simulink model "LF_AC29bus_HVDCdemo_V2_1"  (R2019b)
settings: Solver=FixedStepDiscrete  StartTime=0.0  StopTime=fix(6/Ts)*Ts  FixedStep=Ts  RelTol=1e-3
InitFcn:
  | Ts_avg=150e-6;
  | Ts=50e-6;
  | 
  | %Tc_stab = 1/60/5;
  | %Tc_stab = 2/60;
  | Tc_stab = Ts;
  | 
  | 
  | Ts_avg=150e-6;
  | 
  | Ts=50e-6;
  | 
  | % Rectifier AC side :
  | VLL_nom_R = 735e3; % V
  | Fnom_R = 60;           % Hz
  | 
  | % Inverter AC side :
  | VLL_nom_I = 735e3; % V
  | Fnom_I = 60;           % Hz
  | 
  | % DC :
  | Vdc_nom = 500e3;   % V
  | Idc_nom  = 2000;     % A
undefined symbols (not defined in the file): D1, D11, Delta, test_alpha
libraries: powerlib x223, powerlib_meascontrol x57, simulink x22, sps_avr x7
(part 1 of 10)
Description:
  | Copyright 2008-2012 The MathWorks, Inc.
settings Model: SimulationMode=accelerator  Creator=MathWorks  LastModifiedBy=bhisma
settings DataIOCC: SaveFormat=StructureWithTime  SignalLoggingSaveFormat=ModelDataLogs  SaveOutput=off  SignalLogging=off  DSMLogging=off  SaveTime=off  ReturnWorkspaceOutputs=off
settings OptimizationCC: ExpressionDepthLimit=2147483647  LifeSpan=inf
settings DebuggingCC: UnderspecifiedInitializationDetection=Classic  MergeDetectMultiDrivingBlocksExec=none  SolverPrmCheckMsg=warning  FcnCallInpInsideContextMsg=warning  UnconnectedInputMsg=none  UnconnectedOutputMsg=none  UnconnectedLineMsg=none  StateNameClashWarn=warning  SFUnexpectedBacktrackingDiag=warning  SFNoUnconditionalDefaultTransitionDiag=warning  SFExecutionAtInitializationDiag=none  ArithmeticOperatorsInVariantConditions=warning
settings HardwareCC: ProdBitPerPointer=32  ProdBitPerSizeT=32  ProdBitPerPtrDiffT=32  ProdLargestAtomicFloat=None  ProdIntDivRoundTo=Undefined  ProdEndianess=Unspecified  ProdWordSize=32  ProdHWDeviceType=32-bit Generic
settings ModelReferenceCC: PropagateSignalLabelsOutOfModel=off
settings SFSimCC: SimUseLocalCustomCode=off  CustomCodeUndefinedFunction=UseInterfaceOnly
settings RTWCC: RTWUseLocalCustomCode=off
settings CodeAppCC: StateflowObjectComments=on
settings GRTTargetCC: TargetLangStandard=C89/C90 (ANSI)  GeneratePreprocessorConditionals=Disable all  CombineOutputUpdateFcns=off  GRTInterface=on
settings ConfigComp: CovMetricSettings=dw  CovHtmlReporting=on  CovSaveCumulativeToWorkspaceVar=on  CovSaveSingleToWorkspaceVar=on  CovExternalEMLEnable=off  CovSFcnEnable=off
settings SimscapeCC: SimscapeNormalizeSystem=off

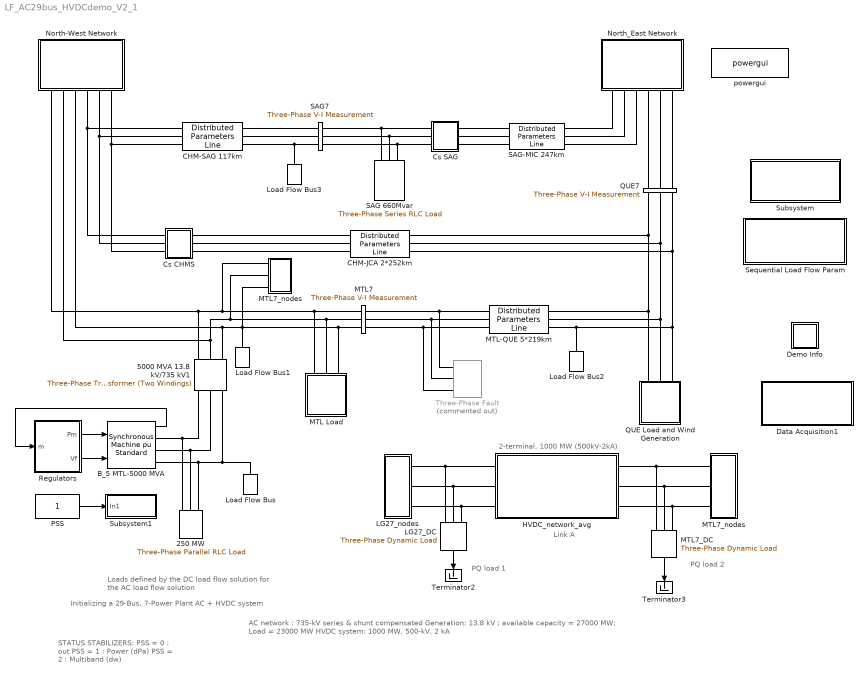
== system LF_AC29bus_HVDCdemo_V2_1 ==
  note: PQ load 1
  note: Link A
  note: AC network :  735-kV series & shunt compensated
      |               Generation: 13.8 kV ; available capacity = 27000 MW;
      |               Load = 23000 MW
      | HVDC system:  1000 MW, 500-kV, 2 kA
  note: Initializing a 29-Bus, 7-Power Plant AC + HVDC system
  note: STATUS STABILIZERS:
      | PSS = 0 :  out
      | PSS = 1 :  Power (dPa)
      | PSS = 2 :  Multiband (dw)
  note: Loads defined by the DC load flow solution
      | for the AC load flow solution
  note: 2-terminal, 1000 MW (500kV-2kA)
  note: PQ load 2
  250 MW : powerlib/Elements/Three-Phase Parallel RLC Load  LConnTagsString=A|B|C  Configuration=Y (grounded)  NominalVoltage=(13800)*1  Vabc=[1e3 1e3 1e3]  Vabcp=[1e3 1e3 1e3]  NominalFrequency=60  UnbalancedPower=off  ActivePower=250000000  InductivePower=0  CapacitivePower=0  Pabc=[10e3 9e3 11e3]  QLabc=[100 90 110]  QCabc=[100 90 110]  Pabcp=[10e3 9e3 11e3]  QLabcp=[100 90 110]  QCabcp=[100 90 110]  Measurements=None  LoadType=constant PQ
      settings: SourceProductName=Simscape Electrical
  5000 MVA 13.8 kV/735 kV1 : powerlib/Elements/Three-Phase Transformer (Two Windings)  Winding1Connection=Delta (D1)  Winding2Connection=Yg  CoreType=Three single-phase transformers  SetSaturation=off  Hysteresis=off  DataFile='basic_model'  SetInitialFlux=off  Measurements=None  UNITS=pu  NominalPower=[ 5000e6 60 ]  Winding1="[ 13.8e3 0.002  0.0]"  Winding2=[ 735e3 0.002 0.12]  Rm=500  Lm=500  L0=0.5  Saturation="[ 0,0  ;  0.005,1.2  ;  1.0,1.4 ]"  InitialFluxes=[ 0.8 , -0.8 , 0.7 ]  BreakLoop=off  DiscreteSolver=Trapezoidal iterative  DataType=off  TransfoNumber=0
      settings: SourceProductName=Simscape Electrical
  B_5 MTL-5000 MVA : powerlib/Machines/Synchronous Machine pu Standard  PresetModel=No  MechanicalLoad=Mechanical power Pm  ShowDetailedParameters=on  RotorType=Salient-pole  Units=per unit standard parameters  MeasurementBus=off  NominalParameters="[5000E6  13800   60 ]"  Reactances1=[ 31 32 33 34 35 36 37 ]  Reactances2=[ 1.305, 0.296, 0.252, 0.474, 0.243, 0.18 ]  dAxisTimeConstants=Short-circuit  qAxisTimeConstants=Open-circuit  TimeConstants1=[]  TimeConstants2=[]  TimeConstants3=[]  TimeConstants4=[]  TimeConstants5=[ 1.01, 0.053, 0.1 ]  TimeConstants6=[]  TimeConstants7=[]  TimeConstants8=[]  StatorResistance=2.8544e-3  Mechanical="[ 3.7 0  32]"  PolePairs=32  InitialConditions=[0 -107.642 0.935091 0.935091 0.935091 -27.7385 -147.738 92.2615 1.11655]  SetSaturation=off  Saturation=[0.6404,0.7127,0.8441,0.9214,0.9956,1.082,1.19,1.316,1.457;0.7,0.7698,0.8872,0.9466,0.9969,1.046,1.1,1.151,1.201]  LoadFlowParameters=[1 4000000000 0 0 0]  TsPowergui=0  TsBlock=-1  IterativeModel=Trapezoidal non iterative  IterativeDiscreteModel=Trapezoidal non iterative  BusType=PV  Pref=4500000000  Qref=0  Qmin=-Inf  Qmax=Inf  PLF=0  QLF=0
      settings: AttributesFormatString=\n\n  SourceProductName=Simscape Electrical
  CHM-JCA 2*252km : powerlib/Elements/Distributed Parameters Line  Phases=3  Frequency=60  Resistance="[0.01273  0.3864]/2"  Inductance="[0.9337e-3  4.1264e-3]/2"  Capacitance=[12.74e-9 7.751e-9]*2  Length=252  x1=[-0.00145 1.55144717799976e-09 0 0;-0.0014 1.46301284014983e-09 0 0;-0.00135 1.3740587008041e-09 0 0;-0.0013 1.28461636494472e-09 0 0;-0.00125 1.19471761100772e-09 0 0;-0.0012 1.10439437959232e-09 0 0;-0.00115 1.01367876211256e-09 0 0;-0.0011 9.22602989395366e-10 0 0;-0.00105 8.31199420229126e-10 0 0;-0.001 7.39500529866733e-10 0 0;-0.00095 6.47538898487297e-10 0 0;-0.0009 5.55347199620561e-10 221588.842093354 -754555.238317053;-0.00085 4.62958188538151e-10 235771.680798918 -750244.605560461;-0.0008 3.70404690615784e-10 249870.750948949 -745667.414467892;-0.00075 2.77719589670567e-10 263881.043210957 -740825.291293546;-0.0007 1.84935816277534e-10 277797.579794812 -735719.956420731;-0.00065 9.20863360695716e-11 291615.416221333 -730353.223750616;-0.0006 -7.95861975116225e-13 305329.643079031 -724727.000057767;-0.00055 -9.36777772538341e-11 318935.387768406 -718843.284312669;-0.0005 -1.86526409264351e-10 332427.816233156 -712704.166971513;-0.00045 -2.79308769329825e-10 345802.134677692 -706311.829233456;-0.0004 -3.71991892319517e-10 359053.591270355 -699668.54226566;-0.00035 -4.64542848361151e-10 372177.477831716 -692776.666396352;-0.0003 -5.56928754540738e-10 385169.13150737 -685638.650276211;-0.00025 -6.49116786585719e-10 398023.936424628 -678257.030008376;-0.0002 -7.41074190527271e-10 410737.325332512 -670634.428247379;-0.00015 -8.32768294337642e-10 423304.78122448 -662773.553267332;-0.0001 -9.2416651953836e-10 435721.838943294 -654677.197999683;-5e-05 -1.01523639277521e-09 447984.086767473 -646348.239040907]  x2=[-0.00145 9.18153078929328e-10 0 0;-0.0014 8.4311629939683e-10 0 0;-0.00135 7.67779964657754e-10 0 0;-0.0013 6.9217084135311e-10 0 0;-0.00125 6.16315793044386e-10 0 0;-0.0012 5.40241770669054e-10 0 0;-0.00115 4.63975802965028e-10 0 0;-0.0011 3.87544986867484e-10 0 0;-0.00105 3.10976477881448e-10 0 0;-0.001 2.34297480433571e-10 0 0;-0.00095 1.57535238206532e-10 0 0;-0.0009 8.07170244594799e-11 -27585.2044281237 -769251.172580331;-0.00085 3.8701323379814e-12 -13081.1063592811 -769634.470687114;-0.0008 -7.29781348231086e-11 1427.63936436365 -769744.321331168;-0.00075 -1.4980047320039e-10 15935.8778545402 -769580.685483081;-0.0007 -2.26569588182836e-10 30438.4544031956 -769143.621281891;-0.00065 -3.03258204069439e-10 44930.2163139378 -768433.284014428;-0.0006 -3.79839073760135e-10 59406.0147327642 -767449.92606014;-0.00055 -4.56284988436573e-10 73860.7064774248 -766193.896801427;-0.0005 -5.32568787229274e-10 88289.1558647705 -764665.642499502;-0.00045 -6.08663366867762e-10 102686.236535437 -762865.706135843;-0.0004 -6.84541691310224e-10 117046.833275214 -760794.72721927;-0.00035 -7.6017680134929e-10 131365.843832462 -758453.441558729;-0.0003 -8.35541824190508e-10 145638.180730909 -755842.681001868;-0.00025 -9.10609983000122e-10 159858.773077217 -752963.373139481;-0.0002 -9.85354606418753e-10 174022.568362636 -749816.540975942;-0.00015 -1.05974913803761e-09 188124.534258145 -746403.302565733;-0.0001 -1.13376714583383e-09 202159.66040241 -742724.870616211;-5e-05 -1.20738233156171e-09 216122.96018194 -738782.552056731]  x3=[-0.00145 4.40533056811722e-12 0 0;-0.0014 4.15180438432733e-12 0 0;-0.00135 3.89680308420899e-12 0 0;-0.0013 3.64041726850993e-12 0 0;-0.00125 3.38273802988964e-12 0 0;-0.0012 3.12385692055464e-12 0 0;-0.00115 2.86386591973038e-12 0 0;-0.0011 2.60285740098147e-12 0 0;-0.00105 2.34092409939181e-12 0 0;-0.001 2.07815907861621e-12 0 0;-0.00095 1.81465569781539e-12 0 0;-0.0009 1.55050757848583e-12 170.673257805867 -126.643772620637;-0.00085 1.28580857119656e-12 173.030090580402 -123.404478428121;-0.0008 1.02065272224447e-12 175.325446587657 -120.121339212024;-0.00075 7.5513424024013e-13 177.558510298572 -116.795521456077;-0.0007 4.89347462635891e-13 179.728488316244 -113.428206807492;-0.00065 2.23386822208262e-13 181.834609657815 -110.020591657131;-0.0006 -4.26531864936143e-14 183.876126028402 -106.57388671443;-0.00055 -3.08678040721427e-13 185.85231208696 -103.089316577243;-0.0005 -5.7459322311118e-13 187.76246570399 -99.5681192967481;-0.00045 -8.40304255264753e-13 189.605908211009 -96.0115459375726;-0.0004 -1.10571673131764e-12 191.381984641671 -92.4208601332958;-0.00035 -1.37073635148089e-12 193.090063964478 -88.7973376374865;-0.0003 -1.63526895554538e-12 194.72953930698 -85.1422658704335;-0.00025 -1.89922055633649e-12 196.299828171393 -81.4569434617318;-0.0002 -2.1624973731073e-12 197.800372641563 -77.7426797888849;-0.00015 -2.42500586485843e-12 199.230639581182 -74.00079451209;-0.0001 -2.68665276357273e-12 200.590120823218 -70.2326171053685;-5e-05 -2.94734510735294e-12 201.87833335046 -66.4394863842103]  x4=[-0.00145 1.03310246252577e-11 0 0;-0.0014 1.01942681995053e-11 0 0;-0.00135 1.00538897988028e-11 0 0;-0.0013 9.90993929892757e-12 0 0;-0.00125 9.76246784480677e-12 0 0;-0.0012 9.61152783234586e-12 0 0;-0.00115 9.45717288981254e-12 0 0;-0.0011 9.29945785878291e-12 0 0;-0.00105 9.13843877465653e-12 0 0;-0.001 8.97417284674726e-12 0 0;-0.00095 8.80671843795713e-12 0 0;-0.0009 8.63613504404022e-12 -600.201413830731 -11265.8928243152;-0.00085 8.46248327246414e-12 -387.75016065453 -11275.2043961627;-0.0008 8.28582482087647e-12 -175.161141692566 -11280.5099415763;-0.00075 8.10622245518387e-12 37.4901111889908 -11281.8075755213;-0.0007 7.92373998725168e-12 250.128044012556 -11279.0968369543;-0.00065 7.73844225223184e-12 462.677107533098 -11272.3786889878;-0.0006 7.55039508552729e-12 675.061784080425 -11261.655518548;-0.00055 7.35966529940095e-12 887.206614390254 -11246.9311355261;-0.0005 7.16632065923764e-12 1099.03622441453 -11228.2107714253;-0.00045 6.9704298594674e-12 1310.47535210146 -11205.5010775019;-0.0004 6.7720624991586e-12 1521.44887413577 -11178.810122402;-0.00035 6.57128905728983e-12 1731.88183262967 -11148.1473892948;-0.0003 6.36818086770898e-12 1941.69946175498 -11113.5237725034;-0.00025 6.16281009378867e-12 2150.82721430717 -11074.9515736341;-0.0002 5.95524970278698e-12 2359.19078819153 -11032.4444972052;-0.00015 5.74557343992252e-12 2566.71615282241 -10986.0176457788;-0.0001 5.53385580217309e-12 2773.32957542592 -10935.6875145941;-5e-05 5.32017201180724e-12 2978.95764723681 -10881.471985707]  x5=0.00142516474882927  V1=ones(3,3)  V2=ones(3,3)  I1=ones(3,3)  I2=ones(3,3)  nHarmo=1  Measurements=None
      settings: AttributesFormatString=\n  SourceProductName=Simscape Electrical
  CHM-SAG 117km : powerlib/Elements/Distributed Parameters Line  Phases=3  Frequency=60  Resistance="[0.01273  0.3864]"  Inductance="[0.9337e-3  4.1264e-3]"  Capacitance=[12.74e-9 7.751e-9]  Length=117  x1=[-0.0007 5.60048893665003e-10 190262.708654527 -766499.647218033;-0.00065 4.66201970309383e-10 204676.244406486 -762777.342481484;-0.0006 3.72189407613588e-10 219017.059663398 -758784.026587206;-0.00055 2.78044607793492e-10 233280.059201887 -754521.118341321;-0.0005 1.83801020048188e-10 247460.175446132 -749990.132334831;-0.00045 8.94921286756525e-11 261552.370268353 -745192.678405489;-0.0004 -4.8485588240748e-12 275551.636778829 -740130.461065832;-0.00035 -9.91875236539387e-11 289453.001104829 -734805.278897577;-0.0003 -1.93491247628942e-10 303251.524157801 -729219.023912592;-0.00025 -2.87726225084993e-10 316942.303388208 -723373.680880673;-0.0002 -3.81858974783315e-10 330520.47452738 -717271.326624366;-0.00015 -4.75856051806162e-10 343981.213315764 -710914.129281082;-0.0001 -5.69684059439648e-10 357319.737216964 -704304.347532766;-5e-05 -6.63309661039432e-10 370531.307116951 -697444.3298034]  x2=[-0.0007 1.29665718229246e-09 231577.82966493 -742341.334076289;-0.00065 1.21438603353582e-09 245528.681687554 -737844.601087074;-0.0006 1.1316834192039e-09 259392.298538689 -733085.715424427;-0.00055 1.04857872314179e-09 273163.754541279 -728066.367897764;-0.0005 9.65101472052274e-10 286838.156762582 -722788.341857361;-0.00045 8.81281325005183e-10 300410.646752602 -717253.512560738;-0.0004 7.97148062899643e-10 313876.402270271 -711463.84650639;-0.00035 7.1273157788307e-10 327230.638996773 -705421.400735097;-0.0003 6.2806186273063e-10 340468.612235386 -699128.32209907;-0.00025 5.43169000188953e-10 353585.618597254 -692586.846499183;-0.0002 4.58083152287871e-10 366576.997672474 -685799.298090569;-0.00015 3.72834549623999e-10 379438.133685921 -678768.088456857;-0.0001 2.87453480619941e-10 392164.457137208 -671495.715753352;-5e-05 2.01970280762963e-10 404751.446424212 -663984.763819445]  x3=[-0.0007 -3.58894977890156e-12 1107.30416704445 -3854.96801229082;-0.00065 -3.60874180811259e-12 1179.76778138122 -3833.41223930973;-0.0006 -3.62725166854264e-12 1251.81222984286 -3810.49447321326;-0.00055 -3.64447278372645e-12 1323.41191537989 -3786.22285657457;-0.0005 -3.66039903508379e-12 1394.54139896497 -3760.60601298349;-0.00045 -3.67502476409338e-12 1465.17540863128 -3733.65304398257;-0.0004 -3.68834477430336e-12 1535.2888484515 -3705.37352583335;-0.00035 -3.70035433317751e-12 1604.85680745432 -3675.77750611398;-0.0003 -3.71104917377676e-12 1673.85456847517 -3644.87550014933;-0.00025 -3.72042549627517e-12 1742.2576169381 -3612.67848727498;-0.0002 -3.72847996930999e-12 1810.04164956569 -3579.1979069363;-0.00015 -3.73520973116532e-12 1877.18258301392 -3544.44565462406;-0.0001 -3.74061239078881e-12 1943.65656242884 -3508.43407764802;-5e-05 -3.74468602864121e-12 2009.43996992207 -3471.17597075003]  x4=[-0.0007 5.91892442933826e-12 20.9018942890144 -1813.92362657518;-0.00065 5.72798036281264e-12 55.0877351514749 -1813.20755055002;-0.0006 5.53500117213857e-12 89.2540036039429 -1811.84725051596;-0.00055 5.3400554219036e-12 123.388560533924 -1809.84320978111;-0.0005 5.14321237540453e-12 157.479278095876 -1807.19614037161;-0.00045 4.94454197003849e-12 191.514044020177 -1803.90698277861;-0.0004 4.74411479245452e-12 225.480765916555 -1799.97690562415;-0.00035 4.54200205347445e-12 259.367375570455 -1795.40730524592;-0.0003 4.33827556279206e-12 293.161833230824 -1790.19980520119;-0.00025 4.13300770345942e-12 326.852131887771 -1784.35625568991;-0.0002 3.92627140616955e-12 360.426301538603 -1777.87873289741;-0.00015 3.71814012334447e-12 393.87241344071 -1770.76953825669;-0.0001 3.50868780303792e-12 427.178584349792 -1763.03119763075;-5e-05 3.29798886266199e-12 460.332980741916 -1754.66646041518]  x5=0.000661683633385019  V1=ones(3,3)  V2=ones(3,3)  I1=ones(3,3)  I2=ones(3,3)  nHarmo=1  Measurements=None
      settings: AttributesFormatString=\n  SourceProductName=Simscape Electrical
  Cs CHMS : Subsystem  mask{Xc=33/2}
      mask prompts: Xc "Condensator Reactance at  60Hz  (ohm):"
      mask help: Series Compensation
      mask init:
      | Cs=1/Xc/(2*pi*60);
      mask Display: disp('Cs')
  Cs SAG : Subsystem  mask{Xc=22}
      mask prompts: Xc "Condensator Reactance at  60Hz  (ohm):"
      mask help: Series Compensation
      mask init:
      | Cs=1/Xc/(2*pi*60);
      mask Display: disp('Cs')
  Data Acquisition1 : Subsystem
      mask Display: disp('Display\n HVDC Waveforms')
  Demo Info : Subsystem
      settings: OpenFcn=web('LF_ACDCdemo_help_V2_1.htm');
      mask Display: disp('?')
  HVDC_network_avg : Subsystem
  LG27_DC : powerlib/Elements/Three-Phase Dynamic Load  NominalVoltage=[ 735e3 60 ]  ActiveReactivePowers=[0 0 ]  PositiveSequence=[1.00802 23.7886]  ExternalControl=off  NpNq="[2  2]"  TimeConstants="[0  0  0  0]"  MinimumVoltage=0.7  Tfilter=1e-4  LoadFlowParameters=[4,0,0,0,0]
      settings: SourceProductName=Simscape Electrical  SourceProductBaseCode=PS
  LG27_nodes : Subsystem
  Load Flow Bus : powerlib/Measurements/Load Flow Bus  LConnTagsString=a  Phases=single  Connectors=on one side  ID=MTL_13.8  Vbase=13.8e3  Vref=1  Vangle=0  VLF=1  VLFb=1  VLFc=1  angleLF=-43.48  angleLFb=0  angleLFc=0
      settings: AttributesFormatString=%<ID>\n%<Vbase>V\n%<VLF>pu\n%<angleLF>deg.  SourceProductName=Simscape Electrical
  Load Flow Bus1 : powerlib/Measurements/Load Flow Bus  LConnTagsString=a  Phases=single  Connectors=on one side  ID=MTL7  Vbase=735e3  Vref=1  Vangle=0  VLF=1.032  VLFb=1  VLFc=1  angleLF=-19.2  angleLFb=0  angleLFc=0
      settings: AttributesFormatString=%<ID>\n%<Vbase>V\n%<VLF>pu\n%<angleLF>deg.  SourceProductName=Simscape Electrical
  Load Flow Bus2 : powerlib/Measurements/Load Flow Bus  LConnTagsString=a  Phases=single  Connectors=on one side  ID=QUE7  Vbase=735e3  Vref=1  Vangle=0  VLF=1.044  VLFb=1  VLFc=1  angleLF=-11.77  angleLFb=0  angleLFc=0
      settings: AttributesFormatString=%<ID>\n%<Vbase>V\n%<VLF>pu\n%<angleLF>deg.  SourceProductName=Simscape Electrical
  Load Flow Bus3 : powerlib/Measurements/Load Flow Bus  LConnTagsString=a  Phases=single  Connectors=on one side  ID=SAG7  Vbase=735e3  Vref=1  Vangle=0  VLF=1.055  VLFb=1  VLFc=1  angleLF=2.357  angleLFb=0  angleLFc=0
      settings: AttributesFormatString=%<ID>\n%<Vbase>V\n%<VLF>pu\n%<angleLF>deg.  SourceProductName=Simscape Electrical
  MTL Load : Subsystem
  MTL-QUE 5*219km : powerlib/Elements/Distributed Parameters Line  Phases=3  Frequency=60  Resistance="[0.01273  0.3864]/5"  Inductance="[0.9337e-3  4.1264e-3]/5"  Capacitance=[12.74e-9 7.751e-9]*5  Length=219  x1=[-0.00125 8.33547483852455e-09 -233824.362483141 -729590.770809669;-0.0012 7.86856650808763e-09 -220031.170302238 -733868.391198433;-0.00115 7.39886251343749e-09 -206159.802094231 -737885.271642205;-0.0011 6.92652973816689e-09 -192215.186290195 -741639.98496249;-0.00105 6.4517359998618e-09 -178202.277345724 -745131.197127525;-0.001 5.97464999047667e-09 -164126.053980644 -748357.66772625;-0.00095 5.49544121639892e-09 -149991.517410091 -751318.250409025;-0.0009 5.01427993822417e-09 -135803.689567603 -754011.893294921;-0.00085 4.53133711026346e-09 -121567.611320858 -756437.639345445;-0.0008 4.04678431980397e-09 -107288.340680669 -758594.626704578;-0.00075 3.5607937261449e-09 -92970.9510039021 -760482.08900498;-0.0007 3.07353799943006e-09 -78620.5291909357 -762099.355640283;-0.00065 2.58519025929904e-09 -64242.1738783087 -763445.852003354;-0.0006 2.09592401337858e-09 -49840.9936271995 -764521.099690445;-0.00055 1.60591309563616e-09 -35422.1051083783 -765324.716671174;-0.0005 1.1153316046176e-09 -20990.6312842786 -765856.417424254;-0.00045 6.24353841590709e-10 -6551.69958883295 -766116.013038938;-0.0004 1.33154248616831e-10 7889.55989427991 -766103.411282142;-0.00035 -3.58092653427551e-10 22328.0162543294 -765818.616631209;-0.0003 -8.49212326857271e-10 36758.5395765212 -765261.730272322;-0.00025 -1.34003027919088e-09 51176.0027646316 -764432.950064554;-0.0002 -1.83037212514701e-09 65575.2833626403 -763332.570469565;-0.00015 -2.32006364860261e-09 79951.2653747147 -761960.982446987;-0.0001 -2.80893086449111e-09 94298.8410828989 -760318.673315513;-5e-05 -3.29680008061852e-09 108612.912861861 -758406.226579756]  x2=[-0.00125 6.16315793044386e-10 -128551.553785848 -758935.218374669;-0.0012 5.40241770669054e-10 -114223.956978345 -761223.405353051;-0.00115 4.63975802965028e-10 -99855.7769428187 -763241.133280166;-0.0011 3.87544986867484e-10 -85452.1186252198 -764987.68526689;-0.00105 3.10976477881448e-10 -71018.0995767636 -766462.440771617;-0.001 2.34297480433571e-10 -56558.8481356889 -767664.875820739;-0.00095 1.57535238206532e-10 -42079.5016051832 -768594.56319481;-0.0009 8.07170244594799e-11 -27585.2044281237 -769251.172580331;-0.00085 3.8701323379814e-12 -13081.1063592811 -769634.470687114;-0.0008 -7.29781348231088e-11 1427.63936436371 -769744.321331168;-0.00075 -1.4980047320039e-10 15935.8778545402 -769580.685483081;-0.0007 -2.26569588182836e-10 30438.4544031956 -769143.621281891;-0.00065 -3.03258204069439e-10 44930.2163139378 -768433.284014428;-0.0006 -3.79839073760135e-10 59406.0147327642 -767449.92606014;-0.00055 -4.56284988436573e-10 73860.7064774248 -766193.896801427;-0.0005 -5.32568787229274e-10 88289.1558647705 -764665.642499502;-0.00045 -6.08663366867762e-10 102686.236535437 -762865.706135843;-0.0004 -6.84541691310224e-10 117046.833275214 -760794.72721927;-0.00035 -7.6017680134929e-10 131365.843832462 -758453.441558729;-0.0003 -8.35541824190508e-10 145638.180730909 -755842.681001868;-0.00025 -9.10609983000122e-10 159858.773077217 -752963.373139481;-0.0002 -9.85354606418753e-10 174022.568362636 -749816.540975942;-0.00015 -1.05974913803761e-09 188124.534258145 -746403.302565733;-0.0001 -1.13376714583383e-09 202159.66040241 -742724.870616211;-5e-05 -1.20738233156171e-09 216122.96018194 -738782.552056731]  x3=[-0.00125 -2.16357456828398e-10 -7879.27372595611 -19699.9030089797;-0.0012 -2.1971766445161e-10 -7506.56090108064 -19844.9149060617;-0.00115 -2.22999807434854e-10 -7131.1810308604 -19982.8759993716;-0.0011 -2.26202719648356e-10 -6753.26748597585 -20113.7372719897;-0.00105 -2.29325263112658e-10 -6372.95453731001 -20237.4522295289;-0.001 -2.32366328402935e-10 -5990.37730824264 -20353.9769166541;-0.00095 -2.35324835043171e-10 -5605.67172664154 -20463.2699326986;-0.0009 -2.38199731890043e-10 -5218.97447656804 -20565.2924463743;-0.00085 -2.4098999750639e-10 -4830.42294971377 -20660.0082095679;-0.0008 -2.43694640524125e-10 -4440.15519658609 -20747.3835702197;-0.00075 -2.46312699996464e-10 -4048.3098774594 -20827.3874842801;-0.0007 -2.4884324573934e-10 -3655.02621310974 -20899.9915267393;-0.00065 -2.51285378661902e-10 -3260.44393535041 -20965.169901727;-0.0006 -2.5363823108595e-10 -2864.70323738584 -21022.8994516766;-0.00055 -2.55900967054221e-10 -2467.94472400164 -21073.1596655542;-0.0005 -2.58072782627401e-10 -2070.30936160842 -21115.9326861448;-0.00045 -2.60152906169758e-10 -1671.93842815704 -21151.2033163981;-0.0004 -2.62140598623301e-10 -1272.97346294327 -21178.959024827;-0.00035 -2.64035153770366e-10 -873.556216319526 -21199.1899499606;-0.0003 -2.65835898484532e-10 -473.828599331667 -21211.8889038473;-0.00025 -2.67542192969775e-10 -73.9326332986557 -21217.0513746094;-0.0002 -2.69153430987789e-10 325.989600646927 -21214.6755280456;-0.00015 -2.7066904007338e-10 725.796012039638 -21204.7622082829;-0.0001 -2.72088481737855e-10 1125.34455156524 -21187.3149374766;-5e-05 -2.73411251660349e-10 1524.49326153012 -21162.3399145588]  x4=[-0.00125 3.18568687534842e-10 -2682.35130404606 -6624.83448605733;-0.0012 3.18771096867668e-10 -2557.00720924975 -6674.21652218367;-0.00115 3.18860248347644e-10 -2430.75462196749 -6721.22724095975;-0.0011 3.18836110299673e-10 -2303.63839914236 -6765.84993970103;-0.00105 3.18698691299888e-10 -2175.70370456306 -6808.06876417513;-0.001 3.18448040172605e-10 -2046.99599281741 -6847.86871423474;-0.00095 3.18084245972977e-10 -1917.56099314252 -6885.23564914712;-0.0009 3.17607437955351e-10 -1787.44469317746 -6920.15629261822;-0.00085 3.17017785527344e-10 -1656.69332262404 -6952.61823750969;-0.0008 3.16315498189657e-10 -1525.35333682163 -6982.60995024709;-0.00075 3.15500825461637e-10 -1393.4714002418 -7010.12077491768;-0.0007 3.14574056792625e-10 -1261.09436990864 -7035.14093705647;-0.00065 3.13535521459116e-10 -1128.26927875071 -7057.66154711897;-0.0006 3.12385588447768e-10 -995.043318890421 -7077.67460363967;-0.00055 3.11124666324307e-10 -861.463824876948 -7095.17299607488;-0.0005 3.09753203088357e-10 -727.578256868456 -7110.15050732909;-0.00045 3.08271686014276e-10 -593.43418376975 -7122.60181596386;-0.0004 3.06680641478026e-10 -459.079266331257 -7132.52249808853;-0.00035 3.04980634770155e-10 -324.561240215397 -7139.90902893198;-0.0003 3.03172269894952e-10 -189.927899036324 -7144.75878409497;-0.00025 3.01256189355845e-10 -55.2270773790884 -7147.07004048258;-0.0002 2.99233073927127e-10 79.4933661957699 -7146.84197691643;-0.00015 2.97103642412077e-10 214.185566156136 -7144.0746744264;-0.0001 2.94868651387571e-10 348.801667004717 -7138.76911622191;-5e-05 2.9252889493528e-10 483.293840281871 -7130.92718734252]  x5=0.00123853603172068  V1=ones(3,3)  V2=ones(3,3)  I1=ones(3,3)  I2=ones(3,3)  nHarmo=1  Measurements=None
      settings: AttributesFormatString=\n  SourceProductName=Simscape Electrical
  MTL7 : powerlib/Measurements/Three-Phase V-I Measurement  VoltageMeasurement=phase-to-ground  SetLabelV=on  LabelV=Vabc_MTL7  Vpu=on  VpuLL=off  CurrentMeasurement=no  SetLabelI=off  LabelI=A1  Ipu=off  Pbase=100e6  Vbase=735e3  OutputType=Magnitude  PhasorSimulation=off  PSBequivalent=0
      settings: SourceProductName=Simscape Electrical
  MTL7_DC : powerlib/Elements/Three-Phase Dynamic Load  NominalVoltage=[735e3 60 ]  ActiveReactivePowers=[0 0 ]  PositiveSequence=[1.03242 -19.1981]  ExternalControl=off  NpNq="[2  2]"  TimeConstants="[0  0  0  0]"  MinimumVoltage=0.7  Tfilter=1e-4  LoadFlowParameters=[4,0,0,0,0]
      settings: SourceProductName=Simscape Electrical  SourceProductBaseCode=PS
  MTL7_nodes : Subsystem
  "MTL7_nodes " : Subsystem
  North-West Network : Subsystem
  North_East Network : Subsystem
  PSS : Constant
  QUE Load and Wind Generation : Subsystem
  QUE7 : powerlib/Measurements/Three-Phase V-I Measurement  VoltageMeasurement=no  SetLabelV=on  LabelV=Vabc_QUE7  Vpu=on  VpuLL=off  CurrentMeasurement=no  SetLabelI=off  LabelI=A1  Ipu=off  Pbase=100e6  Vbase=735e3  OutputType=Magnitude  PhasorSimulation=off  PSBequivalent=0
      settings: SourceProductName=Simscape Electrical
  Regulators : Subsystem
  SAG 660Mvar : powerlib/Elements/Three-Phase Series RLC Load  LConnTagsString=A|B|C  Configuration=Y (grounded)  NominalVoltage=735e3  Vabc=[1e3 1e3 1e3]  Vabcp=[1e3 1e3 1e3]  NominalFrequency=60  UnbalancedPower=off  ActivePower=2200000  InductivePower=660e6  CapacitivePower=0  Pabc=[10e3 9e3 11e3]  QLabc=[100 90 110]  QCabc=[100 90 110]  Pabcp=[10e3 9e3 11e3]  QLabcp=[100 90 110]  QCabcp=[100 90 110]  Measurements=None  LoadType=constant Z
      settings: SourceProductName=Simscape Electrical
  SAG-MIC 247km : powerlib/Elements/Distributed Parameters Line  Phases=3  Frequency=60  Resistance="[0.01273  0.3864]/1"  Inductance="[0.9337e-3  4.1264e-3]/1"  Capacitance=[12.74e-9 7.751e-9]*1  Length=247  x1=[-0.0014 2.27820633104482e-09 4744.33968976524 -768586.454503701;-0.00135 2.20631901232614e-09 19230.170843261 -768360.508638544;-0.0013 2.13364779896803e-09 33709.1696086228 -767861.567943306;-0.00125 2.06021851070656e-09 48176.1916665329 -767089.809689242;-0.0012 1.9860572366182e-09 62626.0969529405 -766045.508078383;-0.00115 1.91119032585053e-09 77053.7514853022 -764729.034146121;-0.0011 1.83564437826043e-09 91454.0291866618 -763140.855629374;-0.00105 1.75944623496338e-09 105821.81370692 -761281.536800407;-0.001 1.68262296879686e-09 120152.000240652 -759151.738266347;-0.00095 1.60520187470153e-09 134439.497340816 -756752.216734471;-0.0009 1.52721046002348e-09 148679.228727725 -754083.824743355;-0.00085 1.44867643474097e-09 162866.13509262 -751147.510359966;-0.0008 1.36962770161925e-09 176995.175895223 -747944.316842824;-0.00075 1.29009234629678e-09 191061.331154614 -744475.382271333;-0.0007 1.2100986273066e-09 205059.603232807 -740741.939141429;-0.00065 1.12967496603617e-09 218985.018610386 -736745.313927677;-0.0006 1.04884993662939e-09 232832.629653577 -732486.926611987;-0.00055 9.6765225583434e-10 246597.516372111 -727968.290179095;-0.0005 8.86110772800385e-10 260274.788167282 -723191.010079009;-0.00045 8.04254458828176e-10 273859.585569546 -718156.783656601;-0.0004 7.22112397076297e-10 287347.081965072 -712867.399548548;-0.00035 6.39713772228161e-10 300732.485310612 -707324.737047838;-0.0003 5.57087860122825e-10 314011.039836096 -701530.765436065;-0.00025 4.74264017353426e-10 327178.027734326 -695487.543283754;-0.0002 3.91271670836926e-10 340228.770837198 -689197.21771896;-0.00015 3.08140307358864e-10 353158.632277832 -682662.023664405;-0.0001 2.24899463096844e-10 365963.018138024 -675884.283043417;-5e-05 1.41578713126471e-10 378637.379080447 -668866.403954967]  x2=[-0.0014 2.20810707032007e-09 102570.511924249 -765608.260365967;-0.00135 2.21038793684379e-09 116982.838636752 -763538.983634143;-0.0013 2.21188346305857e-09 131353.601903715 -761198.425137115;-0.00125 2.21259311761106e-09 145677.695861377 -758587.416464172;-0.0012 2.2125166483644e-09 159950.031227362 -755706.885294263;-0.00115 2.21165408248773e-09 174165.537108872 -752557.855066396;-0.0011 2.2100057264466e-09 188319.162804357 -749141.444616017;-0.00105 2.20757216589407e-09 202405.879598002 -745458.867777492;-0.001 2.20435426546261e-09 216420.682546405 -741511.432952835;-0.00095 2.20035316845693e-09 230358.592256812 -737300.542646845;-0.0009 2.19557029644773e-09 244214.65665627 -732827.692968796;-0.00085 2.19000734876668e-09 257983.952751074 -728094.47310088;-0.0008 2.18366630190258e-09 271661.588375888 -723102.56473358;-0.00075 2.17654940879921e-09 285242.7039319 -717853.741468168;-0.0007 2.16865919805479e-09 298722.474113422 -712349.868186557;-0.00065 2.15999847302362e-09 312096.109622293 -706592.900388718;-0.0006 2.15057031082007e-09 325358.858869498 -700584.883497896;-0.00055 2.14037806122529e-09 338506.009663382 -694327.952133885;-0.0005 2.12942534549702e-09 351532.890883869 -687824.329354606;-0.00045 2.117716055083e-09 364434.874142089 -681076.325866263;-0.0004 2.10525435023836e-09 377207.375424827 -674086.339202365;-0.00035 2.0920446585475e-09 389845.856723194 -666856.852871891;-0.0003 2.07809167335098e-09 402345.827644964 -659390.435476908;-0.00025 2.06340035207799e-09 414702.847009989 -651689.739799966;-0.0002 2.04797591448504e-09 426912.524428128 -643757.501861571;-0.00015 2.03182384080135e-09 438970.521859132 -635596.539948092;-0.0001 2.01494986978179e-09 450872.555153929 -627209.753610437;-5e-05 1.99735999666791e-09 462614.395576763 -618600.122633857]  x3=[-0.0014 -6.4166476964255e-12 -364.997893014476 -3952.48915115888;-0.00135 -6.47904209514277e-12 -290.43459306144 -3958.66659203809;-0.0013 -6.53913452105437e-12 -215.768103080427 -3963.43753752681;-0.00125 -6.59690362360749e-12 -141.024951719794 -3966.80029253083;-0.0012 -6.65232887771508e-12 -66.2316948653227 -3968.75366227929;-0.00115 -6.70539059104827e-12 8.58509379496422 -3969.29695274924;-0.0011 -6.75606991103297e-12 83.3988322123046 -3968.42997091215;-0.00105 -6.8043488315481e-12 158.182939421673 -3966.15302480254;-0.001 -6.85021019932309e-12 232.910844985872 -3962.46692340853;-0.00095 -6.89363772003235e-12 307.555998435881 -3957.37297638438;-0.0009 -6.93461596408455e-12 382.091878704108 -3950.87299358523;-0.00085 -6.9731303721047e-12 456.492003547208 -3942.969284424;-0.0008 -7.00916726010703e-12 530.729938955088 -3933.66465705092;-0.00075 -7.04271382435681e-12 604.779308542791 -3922.96241735581;-0.0007 -7.07375814591952e-12 678.613802921896 -3910.86636779346;-0.00065 -7.10228919489552e-12 752.207189048123 -3897.38080603268;-0.0006 -7.12829683433896e-12 825.533319541805 -3882.51052342936;-0.00055 -7.15177182385938e-12 898.566141977927 -3866.26080332409;-0.0005 -7.17270582290479e-12 971.279708142434 -3848.63741916506;-0.00045 -7.19109139372501e-12 1043.6481832515 -3829.64663245675;-0.0004 -7.20692200401427e-12 1115.64585513051 -3809.29519053523;-0.00035 -7.22019202923211e-12 1187.24714334947 -3787.59032417093;-0.0003 -7.23089675460177e-12 1258.42660831162 -3764.53974499951;-0.00025 -7.23903237678528e-12 1329.15896029198 -3740.15164278199;-0.0002 -7.24459600523482e-12 1399.4190684227 -3714.43468249496;-0.00015 -7.24758566321971e-12 1469.18196962191 -3687.39800125196;-0.0001 -7.24800028852869e-12 1538.42287746299 -3659.0512050571;-5e-05 -7.24583973384736e-12 1607.11719098109 -3629.40436539209]  x4=[-0.0014 1.16657432855998e-11 -154.665030278286 -1728.89575636946;-0.00135 1.1629222765332e-11 -122.050581462933 -1731.50398915601;-0.0013 1.15885704375897e-11 -89.3927686571451 -1733.49702681997;-0.00125 1.15438007459512e-11 -56.7031950263075 -1734.87416124455;-0.0012 1.14949295968749e-11 -23.9934750202759 -1735.63490314045;-0.00115 1.14419743540472e-11 8.7247697531825 -1735.77898221969;-0.0011 1.13849538322139e-11 41.4399146574917 -1735.30634729167;-0.00105 1.13238882904948e-11 74.140336157444 -1734.21716628132;-0.001 1.12587994251861e-11 106.814415948988 -1732.51182616948;-0.00095 1.11897103620517e-11 139.450545087154 -1730.19093285535;-0.0009 1.11166456481068e-11 172.037128110661 -1727.25531094129;-0.00085 1.10396312428964e-11 204.562587161726 -1723.70600343978;-0.0008 1.09586945092719e-11 237.015366099621 -1719.54427140287;-0.00075 1.08738642036694e-11 269.383934606517 -1714.77159347416;-0.0007 1.07851704658924e-11 301.656792284151 -1709.38966536336;-0.00065 1.06926448084039e-11 333.822472739861 -1703.40039924393;-0.0006 1.05963201051291e-11 365.869547660541 -1696.80592307358;-0.00055 1.04962305797767e-11 397.786630873069 -1689.60857983831;-0.0005 1.03924117936783e-11 429.562382389756 -1681.81092671989;-0.00045 1.02849006331543e-11 461.185512437391 -1673.41573418735;-0.0004 1.01737352964081e-11 492.644785468447 -1664.42598501262;-0.00035 1.00589552799545e-11 523.929024153012 -1654.84487321078;-0.0003 9.94060136458688e-12 555.027113350045 -1644.67580290522;-0.00025 9.81871560088776e-12 585.928004056532 -1633.92238711821;-0.0002 9.69334129428862e-12 616.620717333144 -1622.58844648717;-0.00015 9.5645229896836e-12 647.094348204999 -1610.67800790724;-0.0001 9.43230645560295e-12 677.338069536153 -1598.19530310053;-5e-05 9.29673866795167e-12 707.341135876426 -1585.14476711263]  x5=0.00139688767047948  V1=ones(3,3)  V2=ones(3,3)  I1=ones(3,3)  I2=ones(3,3)  nHarmo=1  Measurements=None
      settings: AttributesFormatString=\n  SourceProductName=Simscape Electrical
  SAG7 : powerlib/Measurements/Three-Phase V-I Measurement  VoltageMeasurement=no  SetLabelV=on  LabelV=Vabc_SAG7  Vpu=on  VpuLL=off  CurrentMeasurement=no  SetLabelI=off  LabelI=Iabc_SAG7  Ipu=off  Pbase=100e6  Vbase=735e3  OutputType=Magnitude  PhasorSimulation=off  PSBequivalent=0
      settings: SourceProductName=Simscape Electrical
  Sequential Load Flow Param : Subsystem  mask(Parameters for the sequential AC-DC load flow algorithm){Set_original=on, Model_network=LF_AC29bus_HVDCdemo_V2_1, DC_max_iter=10, DC_AC_max=10, LFDClink=Link_A, Report=ACDC_report_A.txt, bus_rec=LG27, Load_rec=LG27_DC, bus_inv=MTL7, Load_inv=MTL7_DC, second_link=off, LFDClink_B=Link_B, Report_B=ACDC_report_B.txt, bus_rec_B=LG27, Load_rec_B=North-West Network/LG27_DC_B, bus_inv_B=MTL7, load_inv_B=MTL7_DC_B, Start_LF=off}
      mask prompts: Set_original "Reset original work space"; Model_network "AC-DC network model name"; DC_max_iter "Maximum iterations for DC load flow solution"; DC_AC_max "Maximum sequential AC-DC load flows"; LFDClink "DC link steady-state model name"; Report "DC link load flow report name"; bus_rec "Rectifier AC bus name"; Load_rec "PQ load name (Rectifier)"; bus_inv "Inverter AC bus name"; Load_inv "PQ load name (Inverter)"; second_link "Second DC link present"; LFDClink_B "Second DC link steady-state model name"; Report_B "Second DC link load flow report name"; bus_rec_B "Second rectifier AC bus name"; Load_rec_B "PQ load name (Second rectifier)"; bus_inv_B "Second inverter AC bus name"; load_inv_B "PQ load name (Second inverter)"; Start_LF "Start"
      mask help:
      | The block specifies the parameters used by the script  LF_ACDC_solve_V2_1
      | solving by the sequential algorithm the load flow of an AC network that
      | includes one or two HVDC links.  The script is called by the 'Compute' button.
      mask Help: web('Sequential_LF_param_help.htm');
      mask Callback second_link:
      | mode=get_param(gcb,'second_link');
      | cb = get_param(gcb,'MaskEnables');
      | cb{12}='off';cb{13}='off';cb{14}='off';
      | cb{15}='off';cb{16}='off';cb{17}='off';
      | 
      | if strcmp(mode,'on')
      |  cb{12}='on';     % Second DC link model name
      |  cb{13}='on';     % Second DC link report name
      |  cb{14}='on';     % Second rectifier AC bus ...
      |  cb{15}='on';     % PQ load name (second rectifier)
      |  cb{16}='on';     % Second rectifier AC bus ...
      |  cb{17}='on';     % PQ load name (second inverter)
      | end
      | 
      | set_param(gcb,'MaskEnables',cb);
      mask Callback Start_LF:
      | mode=get_param(gcb,'Start_LF');
      | cb = get_param(gcb,'MaskEnables');
      | cb{17}='on';
      | 
      | if strcmp(mode,'on')
      | 
      |  %LF_ACDC_solve_V2b
      |  10
      | end
      | 
      | set_param(gcb,'start_LF','off');
      mask DialogControl Container8 Prompt: Sequential Load flow
      mask DialogControl Execute_LF Prompt: Compute
      mask DialogControl Execute_LF Callback:
      | clear cb mode;
      | eval('LF_ACDC_solve_V2_1');
      mask DialogControl Container6 Prompt: DC link
      mask DialogControl Container29 Prompt: Second DC link
      mask Display: disp('Sequential AC-DC\nload flow\nparameters')
  Subsystem : Subsystem
      mask Display: disp('Display\n AC Waveforms')
  Subsystem1 : Subsystem
      mask Display: disp('PSS_select')
  Terminator2 : Terminator
  Terminator3 : Terminator
  Three-Phase Fault : powerlib/Elements/Three-Phase Fault  Commented=on  InitialStates=0  FaultA=on  FaultB=on  FaultC=on  GroundFault=on  SwitchTimes=[2 2.1]  External=off  SwitchStatus=NaN  FaultResistance=1.0  GroundResistance=0.001  SnubberResistance=1e6  SnubberCapacitance=inf  Measurements=None
      settings: SourceProductName=Simscape Electrical
  powergui : powerlib/powergui  Priority=1  SimulationMode=Discrete  SampleTime=Ts  frequency=60  Iterations=50  frequencyindice=60  Pbase=1e+008  ErrMax=0.0001  UnitsV=kV  UnitsW=MW  buscounter=0  FunctionMessages=off  echomessages=off  EnableUseOfTLC=off  CurrentSourceSwitches=off  DisableSnubberDevices=off  DisableRonSwitches=off  DisableVfSwitches=off  DisplayEquations=off  AutomaticDiscreteSolvers=off  SolverType=Tustin  Interpol=off  ExternalGateDelay=off  methode=off  Ts=10  x0status=blocks  SPID=off  SwTol=0  HookPort=off  NonlinearTolerance=1e-4  nMaxIteration=100  ContinueOnMaxIteration=off  RestoreLinks=warning  ResistiveCurrentMeasurement=off  Frange=[57:0.1:63]  Ylog=off  Xlog=on  ShowGrid=on  save=on  variable=ZData  structure=Vabc_R  ZoomFFT=off  StartTime=4  cycles=3  DisplayStyle=1  fundamental=60  FreqAxis=off  MaxFrequency=500  frequencyindicesteady=1  RmsSteady=1  display=off
      settings: SourceProductName=Simscape Electrical
  wires:
  Regulators/1(Pm) -> B_5 MTL-5000 MVA/1
  Regulators/2(Vf) -> B_5 MTL-5000 MVA/2
  B_5 MTL-5000 MVA/1 -> Regulators/1(m)
  PSS/1 -> Subsystem1/1(In1)
  LG27_DC/1 -> Terminator2/1
  MTL7_DC/1 -> Terminator3/1
  connections:
  QUE Load and Wind Generation/LConn3 -- CHM-JCA 2*252km/RConn3 -- QUE7/LConn3 -- Load Flow Bus2/LConn1 -- MTL-QUE 5*219km/RConn3
  MTL7/RConn1 -- Three-Phase Fault/LConn1 -- MTL-QUE 5*219km/LConn1
  MTL7/RConn2 -- Three-Phase Fault/LConn2 -- MTL-QUE 5*219km/LConn2
  MTL7/RConn3 -- Three-Phase Fault/LConn3 -- MTL-QUE 5*219km/LConn3
  250 MW/LConn1 -- B_5 MTL-5000 MVA/RConn1 -- 5000 MVA 13.8 kV/735 kV1/LConn1
  250 MW/LConn2 -- B_5 MTL-5000 MVA/RConn2 -- 5000 MVA 13.8 kV/735 kV1/LConn2
  5000 MVA 13.8 kV/735 kV1/LConn3 -- Load Flow Bus/LConn1 -- B_5 MTL-5000 MVA/RConn3 -- 250 MW/LConn3
  MTL7/LConn3 -- MTL Load/LConn3 -- Load Flow Bus1/LConn1 -- "MTL7_nodes "/LConn3 -- North-West Network/RConn3 -- 5000 MVA 13.8 kV/735 kV1/RConn3
  MTL-QUE 5*219km/RConn2 -- QUE Load and Wind Generation/LConn2 -- CHM-JCA 2*252km/RConn2 -- QUE7/LConn2
  MTL-QUE 5*219km/RConn1 -- QUE Load and Wind Generation/LConn1 -- CHM-JCA 2*252km/RConn1 -- QUE7/LConn1
  MTL7/LConn2 -- MTL Load/LConn2 -- North-West Network/RConn2 -- 5000 MVA 13.8 kV/735 kV1/RConn2 -- "MTL7_nodes "/LConn2
  Cs SAG/LConn1 -- SAG7/RConn1 -- SAG 660Mvar/LConn1
  Cs SAG/LConn2 -- SAG7/RConn2 -- SAG 660Mvar/LConn2
  Cs SAG/LConn3 -- SAG7/RConn3 -- SAG 660Mvar/LConn3
  Load Flow Bus3/LConn1 -- CHM-SAG 117km/RConn3 -- SAG7/LConn3
  Cs CHMS/LConn1 -- CHM-SAG 117km/LConn1 -- North-West Network/RConn4
  Cs CHMS/LConn2 -- CHM-SAG 117km/LConn2 -- North-West Network/RConn5
  Cs CHMS/LConn3 -- CHM-SAG 117km/LConn3 -- North-West Network/RConn6
  Cs SAG/RConn1 -- SAG-MIC 247km/LConn1
  Cs SAG/RConn3 -- SAG-MIC 247km/LConn3
  Cs CHMS/RConn3 -- CHM-JCA 2*252km/LConn3
  Cs CHMS/RConn2 -- CHM-JCA 2*252km/LConn2
  Cs CHMS/RConn1 -- CHM-JCA 2*252km/LConn1
  Cs SAG/RConn2 -- SAG-MIC 247km/LConn2
  SAG7/LConn2 -- CHM-SAG 117km/RConn2
  SAG7/LConn1 -- CHM-SAG 117km/RConn1
  SAG-MIC 247km/RConn1 -- North_East Network/LConn1
  SAG-MIC 247km/RConn2 -- North_East Network/LConn2
  SAG-MIC 247km/RConn3 -- North_East Network/LConn3
  QUE7/RConn1 -- North_East Network/LConn4
  QUE7/RConn2 -- North_East Network/LConn5
  QUE7/RConn3 -- North_East Network/LConn6
  LG27_nodes/LConn1 -- HVDC_network_avg/LConn1 -- LG27_DC/LConn1
  LG27_nodes/LConn2 -- HVDC_network_avg/LConn2 -- LG27_DC/LConn2
  LG27_nodes/LConn3 -- HVDC_network_avg/LConn3 -- LG27_DC/LConn3
  MTL7_nodes/LConn1 -- HVDC_network_avg/RConn1 -- MTL7_DC/LConn1
  MTL7_nodes/LConn2 -- HVDC_network_avg/RConn2 -- MTL7_DC/LConn2
  MTL7_nodes/LConn3 -- HVDC_network_avg/RConn3 -- MTL7_DC/LConn3
  MTL7/LConn1 -- North-West Network/RConn1 -- 5000 MVA 13.8 kV/735 kV1/RConn1 -- "MTL7_nodes "/LConn1 -- MTL Load/LConn1

== system LF_AC29bus_HVDCdemo_V2_1/Cs CHMS ==
  note: B
  Ca : powerlib/Elements/Series RLC Branch  LConnTagsString=__new0  RConnTagsString=__new0  BranchType=C  Resistance=1.0  Inductance=1.0  SetiL0=off  InitialCurrent=0  Capacitance=Cs  Setx0=off  InitialVoltage=0  Measurements=None
      settings: SourceProductName=Simscape Electrical
  Cb : powerlib/Elements/Series RLC Branch  LConnTagsString=__new0  RConnTagsString=__new0  BranchType=C  Resistance=1.0  Inductance=1.0  SetiL0=off  InitialCurrent=0  Capacitance=Cs  Setx0=off  InitialVoltage=0  Measurements=None
      settings: SourceProductName=Simscape Electrical
  Cc : powerlib/Elements/Series RLC Branch  LConnTagsString=__new0  RConnTagsString=__new0  BranchType=C  Resistance=1.0  Inductance=1.0  SetiL0=off  InitialCurrent=0  Capacitance=Cs  Setx0=off  InitialVoltage=0  Measurements=None
      settings: SourceProductName=Simscape Electrical
  A : PMIOPort  Side=Left
  B : PMIOPort  Port=2  Side=Left
  C : PMIOPort  Port=3  Side=Left
  "A " : PMIOPort  Port=4  Side=Right
  "B " : PMIOPort  Port=5  Side=Right
  "C " : PMIOPort  Port=6  Side=Right
  connections:
  Cc/RConn1 -- "C "/RConn1
  C/RConn1 -- Cc/LConn1
  Cb/RConn1 -- "B "/RConn1
  B/RConn1 -- Cb/LConn1
  Ca/RConn1 -- "A "/RConn1
  A/RConn1 -- Ca/LConn1

== system LF_AC29bus_HVDCdemo_V2_1/Cs SAG ==
  note: B
  Ca : powerlib/Elements/Series RLC Branch  LConnTagsString=__new0  RConnTagsString=__new0  BranchType=C  Resistance=1.0  Inductance=1.0  SetiL0=off  InitialCurrent=0  Capacitance=Cs  Setx0=off  InitialVoltage=0  Measurements=None
      settings: SourceProductName=Simscape Electrical
  Cb : powerlib/Elements/Series RLC Branch  LConnTagsString=__new0  RConnTagsString=__new0  BranchType=C  Resistance=1.0  Inductance=1.0  SetiL0=off  InitialCurrent=0  Capacitance=Cs  Setx0=off  InitialVoltage=0  Measurements=None
      settings: SourceProductName=Simscape Electrical
  Cc : powerlib/Elements/Series RLC Branch  LConnTagsString=__new0  RConnTagsString=__new0  BranchType=C  Resistance=1.0  Inductance=1.0  SetiL0=off  InitialCurrent=0  Capacitance=Cs  Setx0=off  InitialVoltage=0  Measurements=None
      settings: SourceProductName=Simscape Electrical
  A : PMIOPort  Side=Left
  B : PMIOPort  Port=2  Side=Left
  C : PMIOPort  Port=3  Side=Left
  "A " : PMIOPort  Port=4  Side=Right
  "B " : PMIOPort  Port=5  Side=Right
  "C " : PMIOPort  Port=6  Side=Right
  connections:
  A/RConn1 -- Ca/LConn1
  Ca/RConn1 -- "A "/RConn1
  B/RConn1 -- Cb/LConn1
  Cb/RConn1 -- "B "/RConn1
  C/RConn1 -- Cc/LConn1
  Cc/RConn1 -- "C "/RConn1

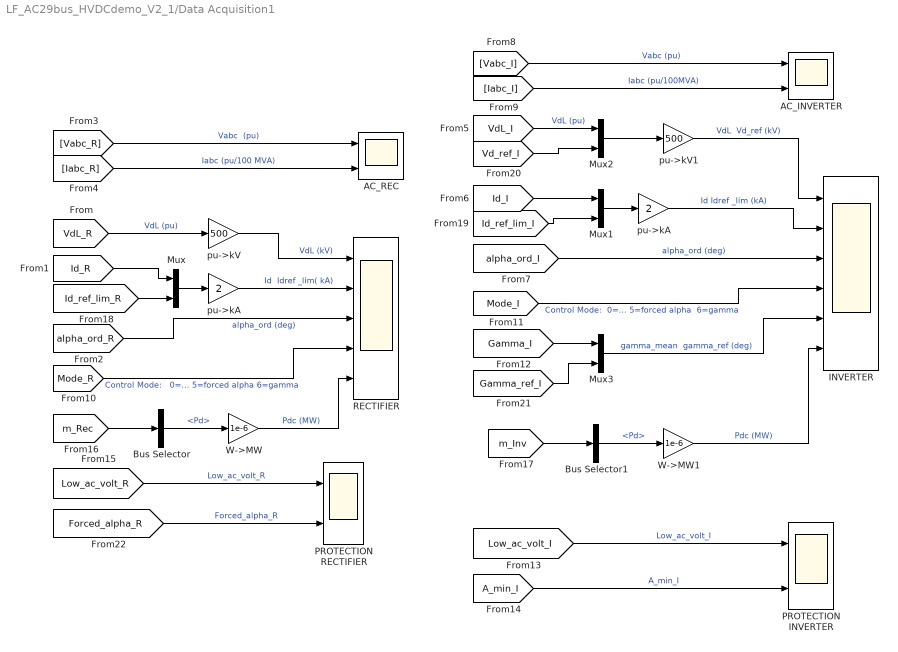
== system LF_AC29bus_HVDCdemo_V2_1/Data Acquisition1 ==
  AC_INVERTER : Scope  NumInputPorts=2
  AC_REC : Scope  NumInputPorts=2
  Bus Selector : BusSelector  OutputSignals=Pd
  Bus Selector1 : BusSelector  OutputSignals=Pd
  INVERTER : Scope  NumInputPorts=6
  Mux{,1..3} (4 alike) : Mux  Inputs=2
  PROTECTION INVERTER : Scope  NumInputPorts=2
  PROTECTION RECTIFIER : Scope  NumInputPorts=2
  RECTIFIER : Scope  NumInputPorts=5
  W->MW : Gain  Gain=1e-6
  W->MW1 : Gain  Gain=1e-6
  pu->kA : Gain  Gain=2
  "pu->kA  " : Gain  Gain=2
  pu->kV : Gain  Gain=500
  pu->kV1 : Gain  Gain=500
  wires:
  [Gamma_ref_I] -> Mux3/2
  [Forced_alpha_R] -> PROTECTION RECTIFIER/2  "Forced_alpha_R"
  Mux3/1 -> INVERTER/5  "gamma_mean  gamma_ref (deg)"
  [Gamma_I] -> Mux3/1
  [Vd_ref_I] -> Mux2/2
  Mux2/1 -> pu->kV1/1
  [VdL_I] -> Mux2/1  "VdL (pu)"
  [Mode_I] -> INVERTER/4  "Control Mode:  0=blocked  1=current  2=voltage  3=alpha min  4=alpha max  5=forced alpha  6=gamma"
  Mux1/1 -> "pu->kA  "/1
  [Id_ref_lim_I] -> Mux1/2
  [Id_I] -> Mux1/1
  [Id_ref_lim_R] -> Mux/2
  [Id_R] -> Mux/1
  Mux/1 -> pu->kA/1
  [Low_ac_volt_R] -> PROTECTION RECTIFIER/1  "Low_ac_volt_R"
  [A_min_I] -> PROTECTION INVERTER/2  "A_min_I"
  [Low_ac_volt_I] -> PROTECTION INVERTER/1  "Low_ac_volt_I"
  [Vabc_R] -> AC_REC/1  "Vabc  (pu)"
  [Iabc_R] -> AC_REC/2  "Iabc (pu/100 MVA)"
  [VdL_R] -> pu->kV/1  "VdL (pu)"
  [alpha_ord_R] -> RECTIFIER/3  "alpha_ord (deg)"
  [Vabc_I] -> AC_INVERTER/1  "Vabc (pu)"
  [Iabc_I] -> AC_INVERTER/2  "Iabc (pu/100MVA)"
  [alpha_ord_I] -> INVERTER/3  "alpha_ord (deg)"
  [Mode_R] -> RECTIFIER/4  "Control Mode:   0=blocked  1=current 2=voltage 3=alpha min  4=alpha max 5=forced alpha 6=gamma"
  [m_Rec] -> Bus Selector/1
  Bus Selector/1 -> W->MW/1  "<Pd>"
  W->MW/1 -> RECTIFIER/5  "Pdc (MW)"
  [m_Inv] -> Bus Selector1/1
  Bus Selector1/1 -> W->MW1/1  "<Pd>"
  W->MW1/1 -> INVERTER/6  "Pdc (MW)"
  pu->kV/1 -> RECTIFIER/1  "VdL (kV)"
  pu->kV1/1 -> INVERTER/1  "VdL  Vd_ref (kV)"
  pu->kA/1 -> RECTIFIER/2  "Id  Idref _lim( kA)"
  "pu->kA  "/1 -> INVERTER/2  "Id Idref _lim (kA)"

== system LF_AC29bus_HVDCdemo_V2_1/Demo Info ==
